simulink model "MMS_ESC_sliding_mode"  (R2019b)
settings: Solver=VariableStepAuto  StartTime=par.sym.TStart  StopTime=par.sym.TStop  FixedStep=par.sym.max_dt  MaxStep=par.sym.max_dt  RelTol=1e-3
undefined symbols (not defined in the file): B, b, beta_K, k, K_0, k_K, m, N_delay, par, rho_K, T_tran, W_K, w_wav
libraries: simulink x1
settings Model: Creator=Vitù  LastModifiedBy=User
settings SolverCC: AutoInsertRateTranBlk=on
settings DataIOCC: SaveFormat=Array  SaveOutput=off  SignalLogging=off  DSMLogging=off  ReturnWorkspaceOutputs=off  TimeSaveName=TIME  OutputSaveName=Yout  OutputOption=SpecifiedOutputTimes  OutputTimes=[par.sym.TStart:par.sym.Outputdt:par.sym.TStop]
settings OptimizationCC: ExpressionDepthLimit=2147483647  LifeSpan=inf
settings DebuggingCC: UnderspecifiedInitializationDetection=Classic  MergeDetectMultiDrivingBlocksExec=none  SolverPrmCheckMsg=warning  AllowSymbolicDim=off  StateNameClashWarn=warning  SFUnexpectedBacktrackingDiag=warning  SFNoUnconditionalDefaultTransitionDiag=warning  SFExecutionAtInitializationDiag=none  ArithmeticOperatorsInVariantConditions=warning
settings HardwareCC: ProdBitPerPointer=32  ProdBitPerSizeT=32  ProdBitPerPtrDiffT=32  ProdLargestAtomicFloat=None  ProdIntDivRoundTo=Undefined  ProdEndianess=Unspecified  ProdWordSize=32  ProdHWDeviceType=32-bit Generic
settings ModelReferenceCC: PropagateSignalLabelsOutOfModel=off
settings SFSimCC: SimUseLocalCustomCode=off  CustomCodeUndefinedFunction=UseInterfaceOnly
settings RTWCC: RTWUseLocalCustomCode=off
settings CodeAppCC: StateflowObjectComments=on
settings GRTTargetCC: TargetLangStandard=C89/C90 (ANSI)  GeneratePreprocessorConditionals=Disable all
settings ConfigComp: CovMetricSettings=dw  CovHtmlReporting=on  CovSaveCumulativeToWorkspaceVar=on  CovSaveSingleToWorkspaceVar=on  CovExternalEMLEnable=off  CovSFcnEnable=off
settings SimscapeCC: SimscapeNormalizeSystem=off
settings ConfigurationSet: Description=SimMechanics 2G

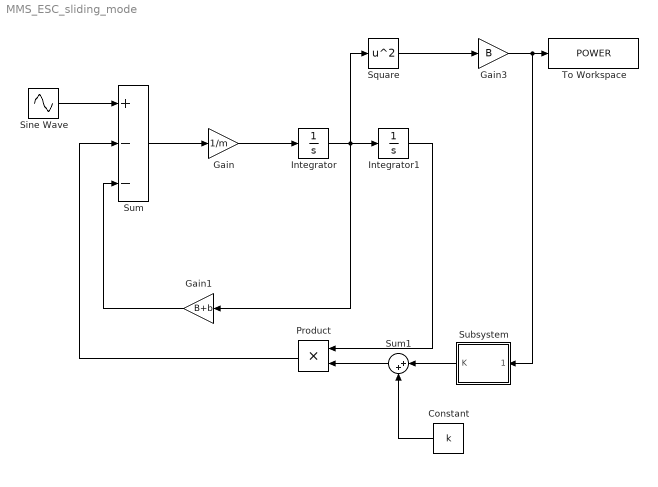
== system MMS_ESC_sliding_mode ==
  Constant : Constant  Value=k
  Gain : Gain  Gain=1/m
  Gain1 : Gain  Gain=B+b
  Gain3 : Gain  Gain=B
  Integrator : Integrator
  Integrator1 : Integrator
  Product : Product
  Sine Wave : Sin  Amplitude=par.H  Frequency=w_wav  SampleTime=0
  Square : Math  Operator=square  SignedPower=off  SaturateOnIntegerOverflow=on
  Subsystem : Subsystem
  Sum : Sum  Inputs=+--
  Sum1 : Sum  Inputs=|++
  To Workspace : ToWorkspace  VariableName=POWER  SampleTime=-1
  wires:
  Product/1 -> Sum/2
  Gain3/1 -> Subsystem/1(POWER), To Workspace/1
  Integrator/1 -> Square/1, Gain1/1, Integrator1/1
  Gain/1 -> Integrator/1
  Gain1/1 -> Sum/3
  Square/1 -> Gain3/1
  Sum/1 -> Gain/1
  Integrator1/1 -> Product/1
  Sine Wave/1 -> Sum/1
  Subsystem/1(K) -> Sum1/1
  Sum1/1 -> Product/2
  Constant/1 -> Sum1/2

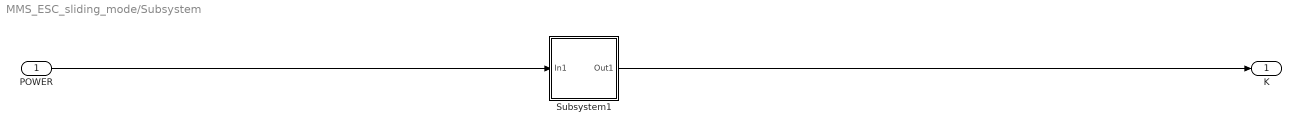
== system MMS_ESC_sliding_mode/Subsystem ==
  POWER : Inport
  Subsystem1 : Subsystem
  K : Outport
  wires:
  POWER/1 -> Subsystem1/1(In1)
  Subsystem1/1(Out1) -> K/1

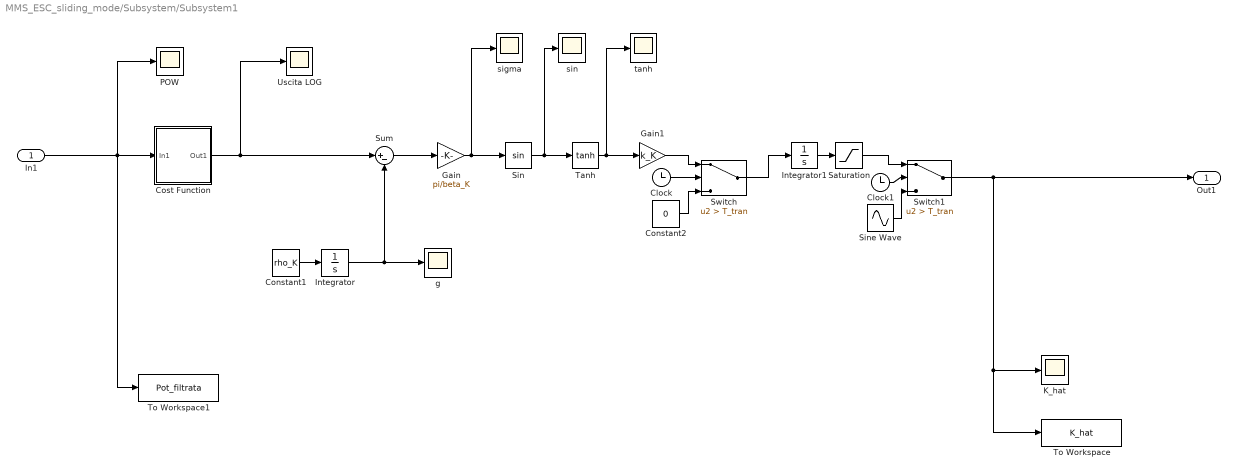
== system MMS_ESC_sliding_mode/Subsystem/Subsystem1 ==
  In1 : Inport
  Clock : Clock
  Clock1 : Clock
  Constant1 : Constant  Value=rho_K
  Constant2 : Constant  Value=0
  Cost Function : Subsystem
  Gain : Gain  Gain=pi/beta_K
  Gain1 : Gain  Gain=k_K
  Integrator : Integrator
  Integrator1 : Integrator  InitialCondition=K_0
  K_hat : Scope
  POW : Scope
  Saturation : Saturate  UpperLimit=inf  LowerLimit=-k
  Sin : Trigonometry
  Sine Wave : Sin  Amplitude=50  Bias=K_0  Frequency=w_wav  SampleTime=0
  Sum : Sum  Inputs=|+-
  Switch : Switch  Criteria=u2 > Threshold  Threshold=T_tran
  Switch1 : Switch  Criteria=u2 > Threshold  Threshold=T_tran
  Tanh : Trigonometry  Operator=tanh
  To Workspace : ToWorkspace  VariableName=K_hat  SampleTime=-1
  To Workspace1 : ToWorkspace  VariableName=Pot_filtrata  SampleTime=-1
  Uscita LOG : Scope
  g : Scope
  sigma : Scope
  sin : Scope
  tanh : Scope
  Out1 : Outport
  wires:
  Integrator/1 -> Sum/2, g/1
  Gain/1 -> sigma/1, Sin/1
  Switch1/1 -> Out1/1, To Workspace/1, K_hat/1
  Sin/1 -> sin/1, Tanh/1
  Tanh/1 -> tanh/1, Gain1/1
  Switch/1 -> Integrator1/1
  Cost Function/1(Out1) -> Uscita LOG/1, Sum/1
  Sine Wave/1 -> Switch1/3
  Clock1/1 -> Switch1/2
  Constant1/1 -> Integrator/1
  Gain1/1 -> Switch/1
  Sum/1 -> Gain/1
  Clock/1 -> Switch/2
  Constant2/1 -> Switch/3
  Integrator1/1 -> Saturation/1
  In1/1 -> To Workspace1/1, POW/1, Cost Function/1(In1)
  Saturation/1 -> Switch1/1

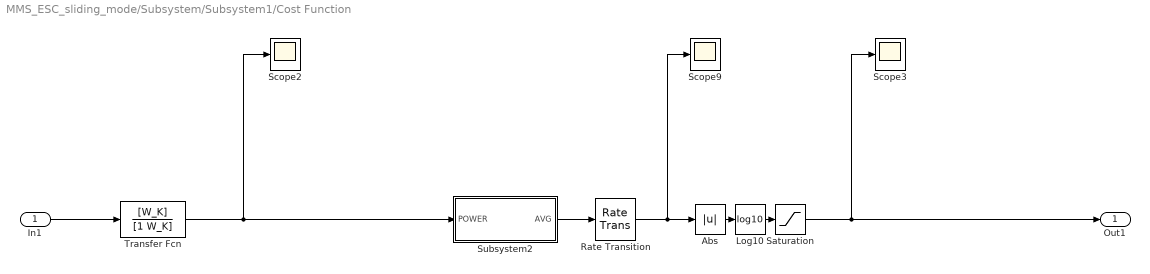
== system MMS_ESC_sliding_mode/Subsystem/Subsystem1/Cost Function ==
  In1 : Inport
  Abs : Abs
  Log10 : Math  Operator=log10  SignedPower=off  SaturateOnIntegerOverflow=on
  Rate Transition : RateTransition
  Saturation : Saturate  UpperLimit=inf  LowerLimit=-40
  Scope2 : Scope
  Scope3 : Scope
  Scope9 : Scope
  Subsystem2 : Subsystem
  Transfer Fcn : TransferFcn  Numerator=[W_K]  Denominator=[1 W_K]
  Out1 : Outport
  wires:
  Subsystem2/1(AVG) -> Rate Transition/1
  Rate Transition/1 -> Abs/1, Scope9/1
  In1/1 -> Transfer Fcn/1
  Transfer Fcn/1 -> Subsystem2/1(POWER), Scope2/1
  Abs/1 -> Log10/1
  Log10/1 -> Saturation/1
  Saturation/1 -> Out1/1, Scope3/1

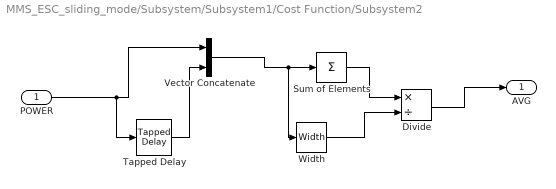
== system MMS_ESC_sliding_mode/Subsystem/Subsystem1/Cost Function/Subsystem2 ==
  POWER : Inport
  Divide : Product  Inputs=*/
  Sum of Elements : Sum  Inputs=+
  Tapped Delay : simulink/Discrete/Tapped Delay  vinit=0  samptime=-1  NumDelays=N_delay  DelayOrder=Oldest  includeCurrent=off
  Vector Concatenate : Concatenate
  Width : Width
  AVG : Outport
  wires:
  POWER/1 -> Tapped Delay/1, Vector Concatenate/1
  Tapped Delay/1 -> Vector Concatenate/2
  Vector Concatenate/1 -> Width/1, Sum of Elements/1
  Sum of Elements/1 -> Divide/1
  Width/1 -> Divide/2
  Divide/1 -> AVG/1
